simulink model "Dahlin_Arduino"  (R2019a)
settings: Solver=FixedStepAuto  StartTime=0.0  StopTime=inf  RelTol=1e-3  EnableMultiTasking=on
libraries: arduinolib x1
settings Model: ExtModeTrigDuration=2  Creator=omare  LastModifiedBy=omare
settings OptimizationCC: EnhancedBackFolding=on  PassReuseOutputArgsAs=Individual arguments  MaxStackSize=64  OptimizeBlockOrder=speed  DifferentSizesBufferReuse=on  OptimizationCustomize=off
settings DebuggingCC: ParameterTunabilityLossMsg=error
settings HardwareCC: ProdBitPerInt=16  ProdBitPerPointer=16  ProdBitPerSizeT=16  ProdBitPerPtrDiffT=16  ProdLargestAtomicFloat=None  ProdWordSize=8  ProdHWDeviceType=Atmel->AVR
settings SFSimCC: MATLABDynamicMemAlloc=off
settings RTWCC: SystemTargetFile=ert.tlc  HardwareBoard=Arduino Uno  TLCOptions=-aInlineSetEventsForThisBaseRateFcn=TLC_FALSE -aSuppressMultiTaskScheduler=TLC_FALSE -aRateBasedStepFcn=1  TemplateMakefile=ert_default_tmf  GenerateReport=on  Toolchain=Arduino AVR  BuildConfiguration=Faster Runs  IncludeHyperlinkInReport=on  LaunchReport=on  GenerateTraceInfo=on  GenerateTraceReport=on  GenerateTraceReportSl=on  GenerateTraceReportSf=on  GenerateTraceReportEml=on
settings CodeAppCC: ForceParamTrailComments=on  IgnoreCustomStorageClasses=off  OperatorAnnotations=on  SimulinkDataObjDesc=on  SFDataObjDesc=on  InsertBlockDesc=on
settings ERTTargetCC: SupportContinuousTime=on  SupportVariableSizeSignals=on  ExtModeStaticAllocSize=250

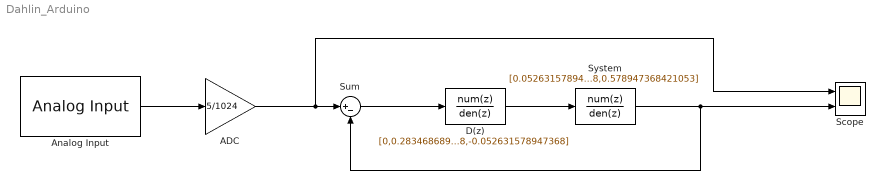
== system Dahlin_Arduino ==
  ADC : Gain  Gain=5/1024  OutDataTypeStr=double
  Analog Input : arduinolib/Analog Input  pinNumber=0  ReadResultsOnly=off  ConversionTriggerSource=Software  ExternalTriggerType=uint32(0)  OutputDataType=uint16  EnableConversionCompleteNotify=off  EnableOuputStatus=off  SampleTime=1  blockPlatform=arduino
  D(z) : DiscreteTransferFcn  Numerator=[0,0.283468689426211,0.208871665892997,0.164113451773069]  Denominator=[0.052631578947368,0.052631578947368,-0.052631578947368,-0.052631578947368]  SampleTime=1
  Scope : Scope  NumInputPorts=2
  Sum : Sum  Inputs=|+-
  System : DiscreteTransferFcn  Numerator=[0.052631578947368,0.105263157894737,0.052631578947368]  Denominator=[1,0.736842105263158,0.578947368421053]  SampleTime=1
  wires:
  Analog Input/1 -> ADC/1
  System/1 -> Scope/2, Sum/2
  ADC/1 -> Sum/1, Scope/1
  D(z)/1 -> System/1
  Sum/1 -> D(z)/1
